simulink library "ReceiveFromPDB"  (R2016b)
settings: Solver=VariableStepAuto  StartTime=0.0  StopTime=10.0  RelTol=1e-3
settings Model: Creator=Nathan  LastModifiedBy=march

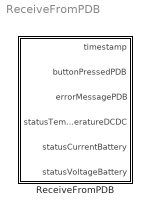
== system ReceiveFromPDB ==
  ReceiveFromPDB : Subsystem

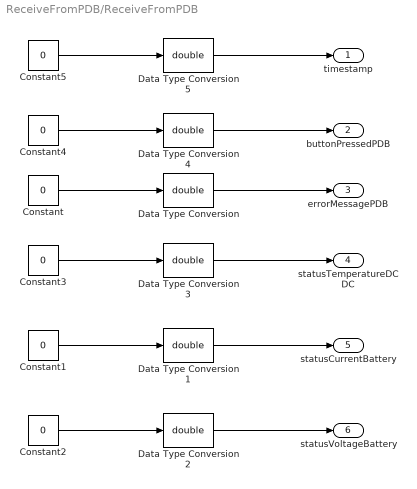
== system ReceiveFromPDB/ReceiveFromPDB ==
  Constant{,1..5} (6 alike) : Constant  Value=0
  Data Type Conversion{,1..5} (6 alike) : DataTypeConversion  OutDataTypeStr=double
  timestamp : Outport
  buttonPressedPDB : Outport  Port=2
  errorMessagePDB : Outport  Port=3
  statusTemperatureDCDC : Outport  Port=4
  statusCurrentBattery : Outport  Port=5
  statusVoltageBattery : Outport  Port=6
  wires:
  Constant5/1 -> Data Type Conversion5/1
  Data Type Conversion5/1 -> timestamp/1
  Constant4/1 -> Data Type Conversion4/1
  Data Type Conversion4/1 -> buttonPressedPDB/1
  Constant3/1 -> Data Type Conversion3/1
  Constant2/1 -> Data Type Conversion2/1
  Constant1/1 -> Data Type Conversion1/1
  Constant/1 -> Data Type Conversion/1
  Data Type Conversion/1 -> errorMessagePDB/1
  Data Type Conversion1/1 -> statusCurrentBattery/1
  Data Type Conversion2/1 -> statusVoltageBattery/1
  Data Type Conversion3/1 -> statusTemperatureDCDC/1
